simulink model "Complementary_Angular_Acceleration_Estimator"  (R2015a)
settings: Solver=ode45  StartTime=0.0  StopTime=2  FixedStep=0.0005  MaxStep=0.001  RelTol=1e-3
libraries: simulink x3, aerolib6dof2 x1
settings Model: Creator=Mitchell  LastModifiedBy=Mitchell

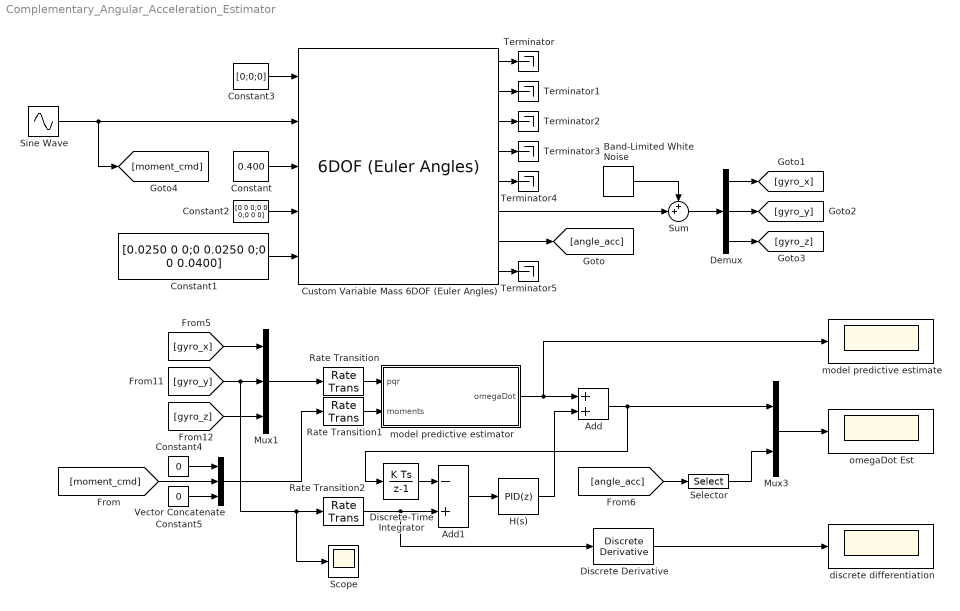
== system Complementary_Angular_Acceleration_Estimator ==
  Add : Sum
  Add1 : Sum  Inputs=-+
  Band-Limited White Noise : simulink/Sources/Band-Limited White Noise  Cov=0.00000001  Ts=0.001  seed=[23341]
  Constant : Constant  Value=0.400
  Constant1 : Constant  Value=[0.0250 0 0;0 0.0250 0;0 0 0.0400]
  Constant2 : Constant  Value=[0 0 0;0 0 0;0 0 0]
  Constant3 : Constant  Value=[0;0;0]
  Constant4 : Constant  Value=0
  Constant5 : Constant  Value=0
  Custom Variable Mass 6DOF (Euler Angles) : aerolib6dof2/6DOF (Euler Angles)  units=Metric (MKS)  mtype=Custom Variable  rep=Euler Angles  xme_0=[0 0 0]  Vm_0=[0 0 0]  eul_0=[0 0 0]  pm_0=[0 0 0]  mass_0=1.0  mass_e=0.5  mass_f=2.0  inertia=eye(3)  inertia_e=eye(3)  inertia_f=2*eye(3)  k_quat=1.0  vre_flag=off
  Demux : Demux  Outputs=3
  Discrete Derivative : simulink/Discrete/Discrete Derivative  gainval=1.0  ICPrevScaledInput=0.0  InputProcessing=Inherited  OutMin=[]  OutMax=[]  OutDataType=fixdt(1, 16)  OutScaling=2^-10  DoSatur=off
  Discrete-Time Integrator : DiscreteIntegrator  InitialConditionSetting=State (most efficient)  SampleTime=0.004
  H(s) : simulink/Continuous/PID Controller  Controller=PID  TimeDomain=Discrete-time  SampleTime=0.004  IntegratorMethod=Forward Euler  FilterMethod=Forward Euler  Form=Parallel  UseFilter=on  ControllerParametersSource=internal  P=14.14  I=100  D=0  N=100  InitialConditionSource=internal  InitialConditionForIntegrator=0  InitialConditionForFilter=0  ExternalReset=none  LimitOutput=off  UpperSaturationLimit=inf  LowerSaturationLimit=-inf  LinearizeAsGain=off  AntiWindupMode=none  Kb=1  TrackingMode=off  Kt=1  PParamMin=[]  PParamMax=[]  IParamMin=[]  IParamMax=[]  DParamMin=[]  DParamMax=[]  NParamMin=[]  NParamMax=[]  KbParamMin=[]  KbParamMax=[]  KtParamMin=[]  KtParamMax=[]  POutMin=[]  POutMax=[]  IOutMin=[]  IOutMax=[]  DOutMin=[]  DOutMax=[]  NOutMin=[]  NOutMax=[]  KbOutMin=[]  KbOutMax=[]  KtOutMin=[]  KtOutMax=[]  IntegratorOutMin=[]  IntegratorOutMax=[]  FilterOutMin=[]  FilterOutMax=[]  SumOutMin=[]  SumOutMax=[]  SumI1OutMin=[]  SumI1OutMax=[]  SumI2OutMin=[]  SumI2OutMax=[]  SumI3OutMin=[]  SumI3OutMax=[]  SumDOutMin=[]  SumDOutMax=[]  SaturationOutMin=[]  SaturationOutMax=[]  IntegratorContinuousStateAttributes=''  IntegratorStateMustResolveToSignalObject=off  IntegratorRTWStateStorageClass=Auto  FilterContinuousStateAttributes=''  FilterStateMustResolveToSignalObject=off  FilterRTWStateStorageClass=Auto  DifferentiatorICPrevScaledInput=0  DifferentiatorOutMin=[]  DifferentiatorOutMax=[]
  Mux1 : Mux  Inputs=3
  Mux3 : Mux  Inputs=2
  Rate Transition : RateTransition  OutPortSampleTime=0.004
  Rate Transition1 : RateTransition  OutPortSampleTime=0.004
  Rate Transition2 : RateTransition  OutPortSampleTime=0.004
  Scope : Scope
  Selector : Selector  InputPortWidth=3  Indices=[2]
  Sine Wave : Sin  Amplitude=0.02  Frequency=6  SampleTime=0
  Sum : Sum  Inputs=++|
  Terminator{,1..5} (6 alike) : Terminator
  Vector Concatenate : Concatenate  NumInputs=3
  discrete differentiation : Scope
  model predictive estimate : Scope
      settings: SaveName=ScopeData2
  model predictive estimator : MATLAB Function  TreatAsAtomicUnit=on
  omegaDot Est : Scope
      settings: SaveName=ScopeData21
  wires:
  [gyro_x] -> Mux1/1
  [gyro_y] -> Rate Transition2/1, Scope/1, Mux1/2
  [gyro_z] -> Mux1/3
  Mux1/1 -> Rate Transition/1
  Add1/1 -> H(s)/1
  Add/1 -> Mux3/1, Discrete-Time Integrator/1
  H(s)/1 -> Add/2
  Mux3/1 -> omegaDot Est/1
  [angle_acc] -> Selector/1
  Selector/1 -> Mux3/2
  Discrete-Time Integrator/1 -> Add1/1
  model predictive estimator/1(omegaDot) -> model predictive estimate/1, Add/1
  Custom Variable Mass 6DOF (Euler Angles)/8 -> Terminator5/1
  Constant/1 -> Custom Variable Mass 6DOF (Euler Angles)/3
  Constant1/1 -> Custom Variable Mass 6DOF (Euler Angles)/5
  Constant2/1 -> Custom Variable Mass 6DOF (Euler Angles)/4
  Constant3/1 -> Custom Variable Mass 6DOF (Euler Angles)/1
  Custom Variable Mass 6DOF (Euler Angles)/7 -> [angle_acc]
  Demux/1 -> [gyro_x]
  Demux/3 -> [gyro_z]
  Demux/2 -> [gyro_y]
  Custom Variable Mass 6DOF (Euler Angles)/1 -> Terminator/1
  Custom Variable Mass 6DOF (Euler Angles)/5 -> Terminator4/1
  Custom Variable Mass 6DOF (Euler Angles)/4 -> Terminator3/1
  Custom Variable Mass 6DOF (Euler Angles)/3 -> Terminator2/1
  Custom Variable Mass 6DOF (Euler Angles)/2 -> Terminator1/1
  [moment_cmd] -> Vector Concatenate/2
  Vector Concatenate/1 -> Rate Transition1/1
  Constant4/1 -> Vector Concatenate/1
  Constant5/1 -> Vector Concatenate/3
  Rate Transition/1 -> model predictive estimator/1(pqr)
  Rate Transition1/1 -> model predictive estimator/2(moments)
  Rate Transition2/1 -> Discrete Derivative/1, Add1/2
  Sine Wave/1 -> [moment_cmd], Custom Variable Mass 6DOF (Euler Angles)/2
  Custom Variable Mass 6DOF (Euler Angles)/6 -> Sum/2
  Sum/1 -> Demux/1
  Band-Limited White Noise/1 -> Sum/1
  Discrete Derivative/1 -> discrete differentiation/1

== matlab function Complementary_Angular_Acceleration_Estimator/model predictive estimator ==
  data: pqr input; omegaDot output; moments input
function omegaDot = fcn(pqr,moments)

Ixx = 0.0250;
Iyy = 0.0250;
Izz = 0.040;
Ixz = 0.000;

omegaDot = ((Izz-Ixx)*pqr(1)*pqr(3) + Ixz*(pqr(3)^2-pqr(1)^2)) / Iyy + moments(2)/Iyy;
